simulink model "testTA"  (R2013a)
settings: Solver=ode45  StartTime=-5  StopTime=10.0  RelTol=1e-3
values from neighbouring files (symbols this model uses):
  FLRThrusters = [6348780.6406300487	6348780.6406304799 6522822.7028749902 6522822.7028749725 			6348780.6406475836 6348780.640630668]    [testTArun.m]
  nbus = 1    [testTArun.m]
  powerAvailableBus = [2568514.3607636942 0 0]    [testTArun.m]
  switchboard2bus = [1 1 1]    [testTArun.m]
  tau_d = [879482.61182011827 1.672023080960795e-07	1.4644506984440428e-05]    [testTArun.m]
  u_old = [-0.021181803858358751 0.021181803851851106	-0.038942104661707069 0.03894210455596573 -0.021181803955349666			0.021181803948799684]    [testTArun.m]
libraries: ThrusterAllocation x1
settings Model: Creator=torstein  LastModifiedBy=torstein
settings DataIOCC: SaveOutput=off  SignalLogging=off  SaveTime=off

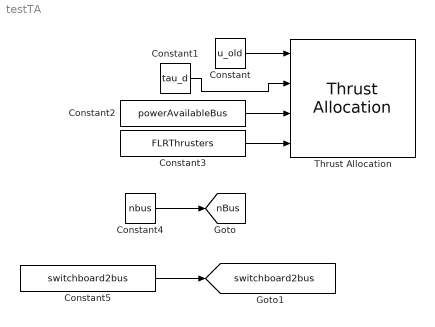
== system testTA ==
  Constant : Constant  Value=u_old
  Constant1 : Constant  Value=tau_d
  Constant2 : Constant  Value=powerAvailableBus
  Constant3 : Constant  Value=FLRThrusters
  Constant4 : Constant  Value=nbus
  Constant5 : Constant  Value=switchboard2bus
  Thrust Allocation : ThrusterAllocation/Thrust Allocation
  tag scope: nBus=global, switchboard2bus=global
  wires:
  Constant/1 -> Thrust Allocation/1
  Constant1/1 -> Thrust Allocation/2
  Constant2/1 -> Thrust Allocation/3
  Constant3/1 -> Thrust Allocation/4
  Constant4/1 -> [nBus]
  Constant5/1 -> [switchboard2bus]
